simulink model "impulse_ex_2b"  (R2024a)
settings: Solver=VariableStepAuto  StartTime=0.0  StopTime=6.23456  RelTol=1e-6  AbsTol=1e-6
undefined symbols (not defined in the file or in its folder): sys
settings Model: DataDictionary=impulseDD.sldd  Creator=grouleau  LastModifiedBy=grouleau

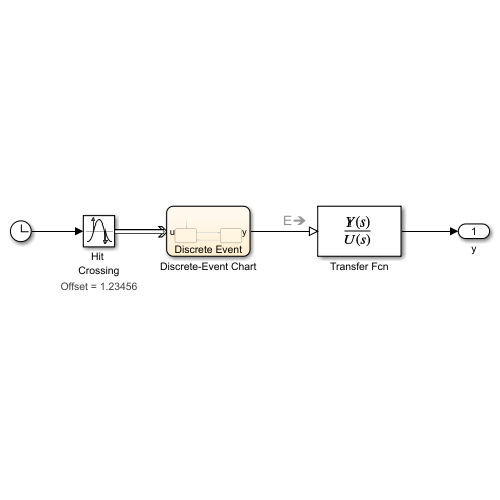
[thumbnail: Simulink's stored preview of the top-level diagram]
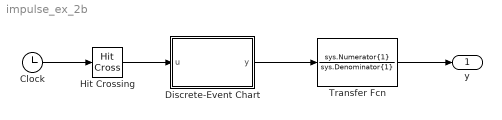
== system impulse_ex_2b ==
  Clock : Clock
  Discrete-Event Chart : Stateflow chart  TreatAsAtomicUnit=on
  Hit Crossing : HitCross  OutputPortMessageModes=m  HitCrossingOffset=1.23456  HitCrossingOutputType=Message
      settings: AttributesFormatString=Offset = %<HitCrossingOffset>
  Transfer Fcn : TransferFcn  Numerator=sys.Numerator{1}  Denominator=sys.Denominator{1}
  y : Outport
  wires:
  Discrete-Event Chart/1(y) -> Transfer Fcn/1
  Transfer Fcn/1 -> y/1
  Hit Crossing/1 -> Discrete-Event Chart/1(u)
  Clock/1 -> Hit Crossing/1

== stateflow chart impulse_ex_2b/Discrete-Event Chart ==
  settings: enableNonTerminalStates=1
  state Off
    en: y=0;
  state On
    en: y = 1/dt;
  (default) -> Off
  Off -> On : u{discard(u)}
  On -> Off : after(dt,sec)
  data: y output; u input; dt parameter
